simulink model "FuelPrimary_harness"  (Simulink 7.7)
settings: Solver=FixedStepDiscrete  SolverMode=SingleTasking  StartTime=0.0  StopTime=100  FixedStep=srate  RelTol=1e-3
InitFcn:
  | if signalbuilder('FuelPrimary_harness/Signal_Builder','activegroup') == 10
  |   CD_FUEL_PRIMARY_FUNCTION.DataType = 'uint8';
  |   CD_FUEL_PRIMARY_FUNCTION.Value = 255;
  | 
  | else
  |   CD_FUEL_PRIMARY_FUNCTION.DataType = 'uint8';
  |   CD_FUEL_PRIMARY_FUNCTION.Value = 0;
  | end
  | 
  | if signalbuilder('FuelPrimary_harness/Signal_Builder','activegroup') == 7
  |   CD_FUEL_PRIMARY_ON_SECONDARY_FAILURE.DataType = 'uint8';
  |   CD_FUEL_PRIMARY_ON_SECONDARY_FAILURE.Value = 0;
  | else
  |   CD_FUEL_PRIMARY_ON_SECONDARY_FAILURE.DataType = 'uint8';
  |   CD_FUEL_PRIMARY_ON_SECONDARY_FAILURE.Value = 255;
  | end
  | 
  | if signalbuilder('FuelPrimary_harness/Signal_Builder','activegroup') == 11
  |   CD_FUEL_PRIMARY_FEEDBACK_FUNCTION.DataType = 'uint8';
  |   CD_FUEL_PRIMARY_FEEDBACK_FUNCTION.Value = 255;
  | elseif signalbuilder('FuelPrimary_harness/Signal_Builder','activegroup') == 10
  |   CD_FUEL_PRIMARY_FEEDBACK_FUNCTION.DataType = 'uint8';
  |   CD_FUEL_PRIMARY_FEEDBACK_FUNCTION.Value = 255;
  | else
  |   CD_FUEL_PRIMARY_FEEDBACK_FUNCTION.DataType = 'uint8';
  |   CD_FUEL_PRIMARY_FEEDBACK_FUNCTION.Value = 0;
  | end
  | 
  | if signalbuilder('FuelPrimary_harness/Signal_Builder','activegroup') == 12
  |   CD_NO_FUEL_WITH_LOW_EOP_FUNCTION.DataType = 'uint8';
  |   CD_NO_FUEL_WITH_LOW_EOP_FUNCTION.Value = 0;
  | elseif signalbuilder('FuelPrimary_harness/Signal_Builder','activegroup') == 13
  |   CD_NO_FUEL_WITH_LOW_EOP_FUNCTION.DataType = 'uint8';
  |   CD_NO_FUEL_WITH_LOW_EOP_FUNCTION.Value = 0;
  | else
  | CD_NO_FUEL_WITH_LOW_EOP_FUNCTION.DataType = 'uint8';
  |   CD_NO_FUEL_WITH_LOW_EOP_FUNCTION.Value = 255;
  | end
  | 
  | 
  | 
  | if signalbuilder('FuelPrimary_harness/Signal_Builder','activegroup') == 13
  |   CD_EOP_FUNCTION.DataType = 'uint8';
  |   CD_EOP_FUNCTION.Value = 1;
  | else
  |   CD_EOP_FUNCTION.DataType = 'uint8';
  |   CD_EOP_FUNCTION.Value = 0;
  | end
undefined symbols (not defined in the file): ACTIVE, ENGINE_CRANKING, ENGINE_NOT_RUNNING, FAILURE, INACTIVE, MXGTW_FUEL_PULL_TIME, NON_FUNCTIONAL, NORMAL, OORL, sigbuilder_block, UNLIMITED
libraries: simulink x2, MX_Library x1
CloseFcn:
  | rtwprivate ssgencode ModelCloseRequest sle_main_controller
settings Model: Creator=smindema  LastModifiedBy=aliebel  RecordCoverage=on  CovPath=Fuel_Primary_Relay/RelaySolenoid  CovMetricSettings=dcmt  CovHTMLOptions=-aTS=1 -bRG=1 -bTC=1 -hTR=0 -nFC=0 -scm=1 -bcm=1 -xEv=0  CovForceBlockReductionOff=off  covSaveCumulativeToWorkspaceVar=off  CovModelRefEnable=off
settings MATStruct: SampleTime=0.01  Offset=0  Priority=[1.0]
settings DataIOCC: LimitDataPoints=off  SaveOutput=off  SaveTime=off
settings OptimizationCC: BlockReduction=off  InlineParams=on  ExpressionFolding=off  StateBitsets=on  DataBitsets=on  UseTempVars=on  InitFltsAndDblsToZero=on  NoFixptDivByZeroProtection=on  EfficientFloat2IntCast=on  OptimizeModelRefInitCode=on
settings DebuggingCC: SaveWithParameterizedLinksMsg=none  MultiTaskDSMMsg=warning  MultiTaskCondExecSysMsg=none  IntegerOverflowMsg=none  ModelReferenceCSMismatchMessage=warning
settings HardwareCC: ProdBitPerInt=16  ProdBitPerPointer=16  ProdIntDivRoundTo=Floor  ProdEndianess=BigEndian  ProdWordSize=16  ProdHWDeviceType=Motorola HC12
settings ModelReferenceCC: ModelReferenceNumInstancesAllowed=Single
settings RTWCC: SystemTargetFile=ert.tlc  GenCodeOnly=on  TemplateMakefile=ert_default_tmf  Description=Real-Time Workshop Embedded Coder (no auto configuration)  GenerateReport=on  RetainRTWFile=on  ProcessScript=ert_make_rtw_hook  IncludeHyperlinkInReport=on  LaunchReport=on  IncludeERTFirstTime=on
settings RTWCC: CustomHeaderCode=|
  | #include "cpp_req_defines.h"
  | #include "hw_fin.h"
  | #include "cdata.h"
settings CodeAppCC: IgnoreCustomStorageClasses=off  DefineNamingRule=UpperCase
settings ERTTargetCC: TargetFcnLib=ansi_tfl_tmw.mat  FunctionExecutionProfile=off  MultiwordLength=2048  GenerateSampleERTMain=on  IncludeMdlTerminateFcn=off  SupportAbsoluteTime=off  SupportNonFinite=off  SupportComplex=off  PurelyIntegerCode=on  ERTCustomFileTemplate=gen_rtw_req_defines_h.tlc  GlobalDataDefinition=InSeparateSourceFile  GlobalDataReference=InSeparateHeaderFile  ConvertIfToSwitch=off

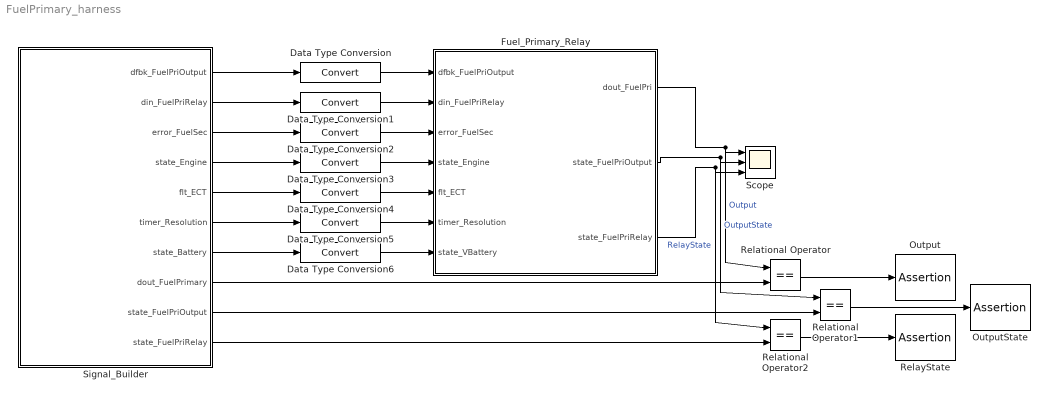
== system FuelPrimary_harness ==
  Data Type Conversion{,1..6} (7 alike) : DataTypeConversion
  Fuel_Primary_Relay : Subsystem  TreatAsAtomicUnit=on
      settings: RTWSystemCode=Function  RTWFcnNameOpts=Use subsystem name
  Output : Assertion  Enabled=off
  OutputState : Assertion  Enabled=off
  Relational Operator : RelationalOperator  Operator===  OutDataTypeStr=boolean
  Relational Operator1 : RelationalOperator  Operator===  OutDataTypeStr=boolean
  Relational Operator2 : RelationalOperator  Operator===  OutDataTypeStr=boolean
  RelayState : Assertion  Enabled=off
  Scope : Scope  NumInputPorts=3
      settings: YMin=0~0~0  YMax=2~10~10  MaxDataPoints=50000
  Signal_Builder : Subsystem  Tag=STV Subsys  LoadFcn=sigbuilder_block('load');  StartFcn=sigbuilder_block('start');  StopFcn=sigbuilder_block('stop');  ClipboardFcn=sigbuilder_block('clipboard');  mask(Sigbuilder block){}
      mask help: Sigbuilder GUI
      mask init:
      | if ~strcmp(get_param(bdroot(gcbh),'SimulationStatus'),'stopped') tuvar = sigbuilder_block('maskInit'); end
      settings: CopyFcn=sigbuilder_block('copy');  DeleteFcn=sigbuilder_block('delete');  ModelCloseFcn=sigbuilder_block('modelClose');  PreSaveFcn=sigbuilder_block('preSave');  NameChangeFcn=sigbuilder_block('namechange');  OpenFcn=sigbuilder_block('open',[55.5 123.75 1080 620.25 ]);  CloseFcn=sigbuilder_block('close');
      mask Display: plot(0,0,100,100,[10,10,40,40,10],[80,20,20,80,80],[40,10],[50,50], [40,27,10],[65,72,56],[40,25,25,10],[28,28,43,43]);
  wires:
  Fuel_Primary_Relay/1(dout_FuelPri) -> Scope/1, Relational Operator/1  "Output"
  Fuel_Primary_Relay/2(state_FuelPriOutput) -> Scope/2, Relational Operator1/1  "OutputState"
  Fuel_Primary_Relay/3(state_FuelPriRelay) -> Scope/3, Relational Operator2/1  "RelayState"
  Relational Operator/1 -> Output/1
  Relational Operator1/1 -> OutputState/1
  Relational Operator2/1 -> RelayState/1
  Signal_Builder/8(dout_FuelPrimary) -> Relational Operator/2
  Signal_Builder/9(state_FuelPriOutput) -> Relational Operator1/2
  Signal_Builder/10(state_FuelPriRelay) -> Relational Operator2/2
  Data Type Conversion/1 -> Fuel_Primary_Relay/1(dfbk_FuelPriOutput)
  Data Type Conversion1/1 -> Fuel_Primary_Relay/2(din_FuelPriRelay)
  Data Type Conversion2/1 -> Fuel_Primary_Relay/3(error_FuelSec)
  Data Type Conversion3/1 -> Fuel_Primary_Relay/4(state_Engine)
  Data Type Conversion4/1 -> Fuel_Primary_Relay/5(flt_ECT)
  Data Type Conversion5/1 -> Fuel_Primary_Relay/6(timer_Resolution)
  Data Type Conversion6/1 -> Fuel_Primary_Relay/7(state_VBattery)
  Signal_Builder/1(dfbk_FuelPriOutput) -> Data Type Conversion/1
  Signal_Builder/2(din_FuelPriRelay) -> Data Type Conversion1/1
  Signal_Builder/3(error_FuelSec) -> Data Type Conversion2/1
  Signal_Builder/4(state_Engine) -> Data Type Conversion3/1
  Signal_Builder/5(flt_ECT) -> Data Type Conversion4/1
  Signal_Builder/6(timer_Resolution) -> Data Type Conversion5/1
  Signal_Builder/7(state_Battery) -> Data Type Conversion6/1

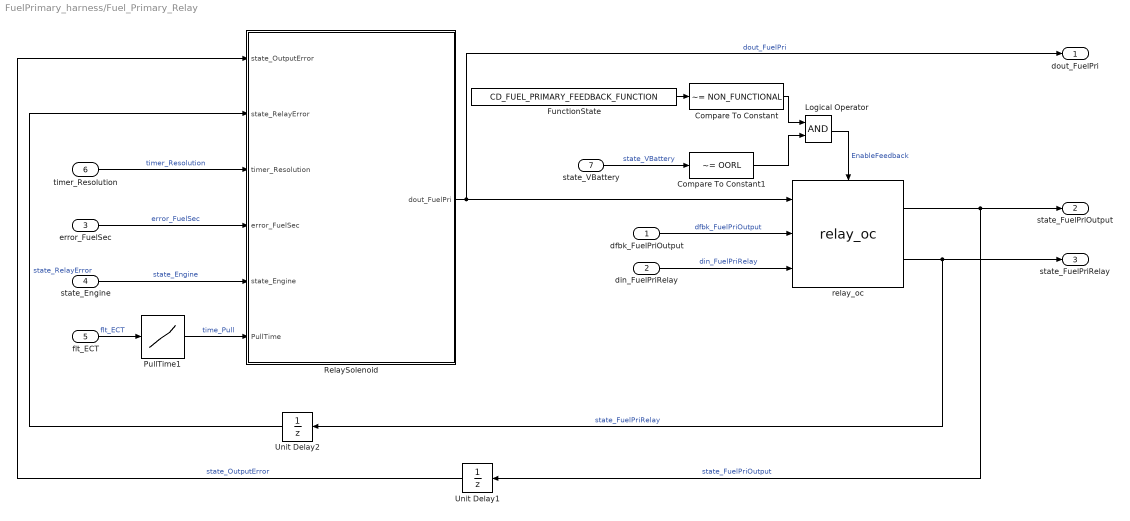
== system FuelPrimary_harness/Fuel_Primary_Relay ==
  dfbk_FuelPriOutput : Inport  OutDataTypeStr=boolean
  din_FuelPriRelay : Inport  Port=2  OutDataTypeStr=boolean
  error_FuelSec : Inport  Port=3  OutDataTypeStr=uint8
  state_Engine : Inport  Port=4
  flt_ECT : Inport  Port=5  OutDataTypeStr=uint16
  timer_Resolution : Inport  Port=6  OutDataTypeStr=uint8
  state_VBattery : Inport  Port=7
  Compare To Constant : simulink/Logic and Bit Operations/Compare To Constant  SystemSampleTime=-1  relop=~=  const=NON_FUNCTIONAL  LogicOutDataTypeMode=boolean  ZeroCross=off
  Compare To Constant1 : simulink/Logic and Bit Operations/Compare To Constant  SystemSampleTime=-1  relop=~=  const=OORL  LogicOutDataTypeMode=boolean  ZeroCross=off
  FunctionState : Constant  Value=CD_FUEL_PRIMARY_FEEDBACK_FUNCTION  OutDataTypeStr=uint8
  Logical Operator : Logic  AllPortsSameDT=off  OutDataTypeStr=boolean
  PullTime1 : Lookup  InputValues=0:8:336  Table=MXGTW_FUEL_PULL_TIME  LookUpMeth=Use Input Nearest  OutDataTypeStr=uint16  RndMeth=Nearest
      settings: AttributesFormatString=input = %<InputValues>\noutput = %<OutputValues>\nlookup = %<LookUpMeth>\nrounding = %<RndMeth>
  RelaySolenoid : Stateflow chart  TreatAsAtomicUnit=on
  Unit Delay1 : UnitDelay  SampleTime=-1
      settings: AttributesFormatString=<initial=%<X0>>\n<tsample=%<SampleTime>>
  Unit Delay2 : UnitDelay  SampleTime=-1
      settings: AttributesFormatString=<initial=%<X0>>\n<tsample=%<SampleTime>>
  relay_oc : MX_Library/relay_oc  SystemSampleTime=-1  ERROR_ON_DB_CNT=CD_FUEL_PRIMARY_DEBOUNCE_ERROR_ON  ERROR_OFF_DB_CNT=CD_FUEL_PRIMARY_DEBOUNCE_ERROR_OFF  NORMAL_DB_CNT=CD_FUEL_PRIMARY_DEBOUNCE_NORMAL
  dout_FuelPri : Outport  OutDataTypeStr=boolean
  state_FuelPriOutput : Outport  Port=2  OutDataTypeStr=uint8
  state_FuelPriRelay : Outport  Port=3  OutDataTypeStr=uint8
  wires:
  timer_Resolution/1 -> RelaySolenoid/3(timer_Resolution)  "timer_Resolution"
  flt_ECT/1 -> PullTime1/1  "flt_ECT"
  state_Engine/1 -> RelaySolenoid/5(state_Engine)  "state_Engine"
  Logical Operator/1 -> relay_oc/Enable  "EnableFeedback"
  Compare To Constant1/1 -> Logical Operator/2
  Compare To Constant/1 -> Logical Operator/1
  state_VBattery/1 -> Compare To Constant1/1  "state_VBattery"
  FunctionState/1 -> Compare To Constant/1
  relay_oc/1 -> Unit Delay1/1, state_FuelPriOutput/1  "state_FuelPriOutput"
  Unit Delay2/1 -> RelaySolenoid/2(state_RelayError)  "state_RelayError"
  Unit Delay1/1 -> RelaySolenoid/1(state_OutputError)  "state_OutputError"
  relay_oc/2 -> Unit Delay2/1, state_FuelPriRelay/1  "state_FuelPriRelay"
  din_FuelPriRelay/1 -> relay_oc/3  "din_FuelPriRelay"
  dfbk_FuelPriOutput/1 -> relay_oc/2  "dfbk_FuelPriOutput"
  RelaySolenoid/1(dout_FuelPri) -> dout_FuelPri/1, relay_oc/1  "dout_FuelPri"
  error_FuelSec/1 -> RelaySolenoid/4(error_FuelSec)  "error_FuelSec"
  PullTime1/1 -> RelaySolenoid/6(PullTime)  "time_Pull"

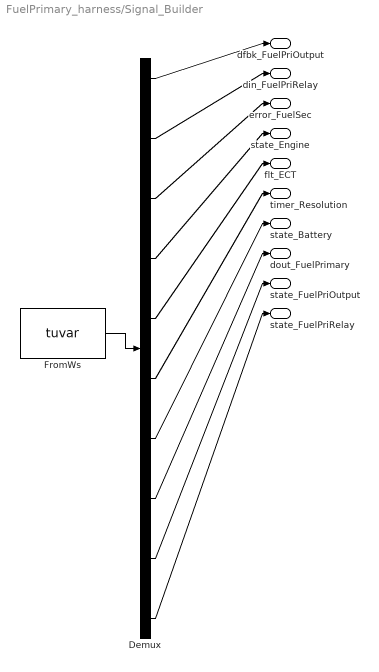
== system FuelPrimary_harness/Signal_Builder ==
  Demux : Demux  Tag=STV Demux  Outputs=10
  FromWs : FromWorkspace  Tag=STV FromWs  VariableName=tuvar  SampleTime=0  SigBuilderData=DataTag0  VnvData=DataTag1
      SigBuilderData=|
      | common.afterFinalStr = 'Extrapolate'
      | common.sampleTime = 0
      | dataSet(1).timeRange = [0 100]
      | dataSet(1).name = 'Normal'
      | dataSet(2).timeRange = [0 100]
      | dataSet(2).name = 'Relay OC'
      | dataSet(3).timeRange = [0 100]
      | dataSet(3).name = 'Output Cont Error'
      | dataSet(4).timeRange = [0 100]
      | dataSet(4).name = 'Relay Error On'
      | dataSet(5).timeRange = [0 100]
      | dataSet(5).name = 'Relay Error Off'
      | dataSet(6).timeRange = [0 100]
      | dataSet(6).name = 'Battery'
      | dataSet(7).timeRange = [0 100]
      | dataSet(7).name = 'SecondaryFuel'
      | dataSet(8).timeRange = [0 100]
      | dataSet(8).name = 'Error ON'
      | dataSet(9).timeRange = [0 100]
      | dataSet(9).name = 'Error OFF'
      | dataSet(10).timeRange = [0 100]
      | dataSet(10).name = 'NONFUNC'
      | dataSet(11).timeRange = [0 100]
      | dataSet(11).name = 'NO FDBK'
      | dataSet(12).timeRange = [0 100]
      | dataSet(12).name = 'Output Error On'
      | dataSet(13).timeRange = [0 100]
      | dataSet(13).name = 'Output Error Off'
      | sbobj.Groups(1).Name = 'Normal'
      | sbobj.Groups(1).Signals(1).Name = 'dfbk_FuelPriOutput'
      | sbobj.Groups(1).Signals(1).XData = [0 20 20 22.2 22.2 60 60 61.4 61.4 100]
      | sbobj.Groups(1).Signals(1).YData = [0 0 1 1 0 0 1 1 0 0]
      | sbobj.Groups(1).Signals(2).Name = 'din_FuelPriRelay'
      | sbobj.Groups(1).Signals(2).XData = [0 20 20 22.2 22.2 60 60 61.4 61.4 100]
      | sbobj.Groups(1).Signals(2).YData = [0 0 1 1 0 0 1 1 0 0]
      | sbobj.Groups(1).Signals(3).Name = 'error_FuelSec'
      | sbobj.Groups(1).Signals(3).XData = [0 100]
      | sbobj.Groups(1).Signals(3).YData = [8 8]
      | sbobj.Groups(1).Signals(4).Name = 'state_Engine'
      | sbobj.Groups(1).Signals(4).XData = [0 20 20 30 30 50 50 60 60 61.2 61.2 62.6 62.6 64.2 64.2 100]
      | sbobj.Groups(1).Signals(4).YData = [1 1 2 2 3 3 1 1 2 2 1 1 2 2 1 1]
      | sbobj.Groups(1).Signals(5).Name = 'flt_ECT'
      | sbobj.Groups(1).Signals(5).XData = [0 49.9 49.9 100]
      | sbobj.Groups(1).Signals(5).YData = [0 0 200 200]
      | sbobj.Groups(1).Signals(6).Name = 'timer_Resolution'
      | sbobj.Groups(1).Signals(6).XData = [0 61.5 61.5 64.8 64.8 100]
      | sbobj.Groups(1).Signals(6).YData = [0 0 1 1 0 0]
      | sbobj.Groups(1).Signals(7).Name = 'state_Battery'
      | sbobj.Groups(1).Signals(7).XData = [0 100]
      | sbobj.Groups(1).Signals(7).YData = [8 8]
      | sbobj.Groups(1).Signals(8).Name = 'dout_FuelPrimary'
      | sbobj.Groups(1).Signals(8).XData = [0 20 20 22.11 22.11 60 60 61.2 61.2 100]
      | sbobj.Groups(1).Signals(8).YData = [0 0 1 1 0 0 1 1 0 0]
      | sbobj.Groups(1).Signals(9).Name = 'state_FuelPriOutput'
      | sbobj.Groups(1).Signals(9).XData = [0 100]
      | sbobj.Groups(1).Signals(9).YData = [8 8]
      | sbobj.Groups(1).Signals(10).Name = 'state_FuelPriRelay'
      | sbobj.Groups(1).Signals(10).XData = [0 100]
      | sbobj.Groups(1).Signals(10).YData = [8 8]
      | sbobj.Groups(2).Name = 'Relay OC'
      | sbobj.Groups(2).Signals(1).Name = 'dfbk_FuelPriOutput'
      | sbobj.Groups(2).Signals(1).XData = [0 10 10 30 30 100]
      | sbobj.Groups(2).Signals(1).YData = [0 0 1 1 0 0]
      | sbobj.Groups(2).Signals(2).Name = 'din_FuelPriRelay'
      | sbobj.Groups(2).Signals(2).XData = [0 100]
      | sbobj.Groups(2).Signals(2).YData = [0 0]
      | sbobj.Groups(2).Signals(3).Name = 'error_FuelSec'
      | sbobj.Groups(2).Signals(3).XData = [0 100]
      | sbobj.Groups(2).Signals(3).YData = [8 8]
      | sbobj.Groups(2).Signals(4).Name = 'state_Engine'
      | sbobj.Groups(2).Signals(4).XData = [0 20 20 30 30 50 50 69.9 100]
      | sbobj.Groups(2).Signals(4).YData = [1 1 2 2 3 3 1 1 1]
      | sbobj.Groups(2).Signals(5).Name = 'flt_ECT'
      | sbobj.Groups(2).Signals(5).XData = [0 100]
      | sbobj.Groups(2).Signals(5).YData = [150 150]
      | sbobj.Groups(2).Signals(6).Name = 'timer_Resolution'
      | sbobj.Groups(2).Signals(6).XData = [0 100]
      | sbobj.Groups(2).Signals(6).YData = [0 0]
      | sbobj.Groups(2).Signals(7).Name = 'state_Battery'
      | sbobj.Groups(2).Signals(7).XData = [0 100]
      | sbobj.Groups(2).Signals(7).YData = [8 8]
      | sbobj.Groups(2).Signals(8).Name = 'dout_FuelPrimary'
      | sbobj.Groups(2).Signals(8).XData = [0 100]
      | sbobj.Groups(2).Signals(8).YData = [0 0]
      | sbobj.Groups(2).Signals(9).Name = 'state_FuelPriOutput'
      | sbobj.Groups(2).Signals(9).XData = [0 10.05 10.05 100]
      | sbobj.Groups(2).Signals(9).YData = [8 8 7 7]
      | sbobj.Groups(2).Signals(10).Name = 'state_FuelPriRelay'
      | sbobj.Groups(2).Signals(10).XData = [0 10.05 100]
      | sbobj.Groups(2).Signals(10).YData = [8 8 8]
      | sbobj.Groups(3).Name = 'Output Cont Error'
      | sbobj.Groups(3).Signals(1).Name = 'dfbk_FuelPriOutput'
      | sbobj.Groups(3).Signals(1).XData = [0 100]
      | sbobj.Groups(3).Signals(1).YData = [0 0]
      | sbobj.Groups(3).Signals(2).Name = 'din_FuelPriRelay'
      | sbobj.Groups(3).Signals(2).XData = [0 20 20 21.61 21.61 60 60 61.61 61.61 100]
      | sbobj.Groups(3).Signals(2).YData = [0 0 1 1 0 0 1 1 0 0]
      | sbobj.Groups(3).Signals(3).Name = 'error_FuelSec'
      | sbobj.Groups(3).Signals(3).XData = [0 100]
      | sbobj.Groups(3).Signals(3).YData = [8 8]
      | sbobj.Groups(3).Signals(4).Name = 'state_Engine'
      | sbobj.Groups(3).Signals(4).XData = [0 20 20 30 30 50 50 60 60 70.1 70.1 80.1 100]
      | sbobj.Groups(3).Signals(4).YData = [1 1 2 2 3 3 1 1 2 2 1 1 1]
      | sbobj.Groups(3).Signals(5).Name = 'flt_ECT'
      | sbobj.Groups(3).Signals(5).XData = [0 100]
      | sbobj.Groups(3).Signals(5).YData = [130 130]
      | sbobj.Groups(3).Signals(6).Name = 'timer_Resolution'
      | sbobj.Groups(3).Signals(6).XData = [0 100]
      | sbobj.Groups(3).Signals(6).YData = [0 0]
      | sbobj.Groups(3).Signals(7).Name = 'state_Battery'
      | sbobj.Groups(3).Signals(7).XData = [0 100]
      | sbobj.Groups(3).Signals(7).YData = [8 8]
      | sbobj.Groups(3).Signals(8).Name = 'dout_FuelPrimary'
      | sbobj.Groups(3).Signals(8).XData = [0 20 20 21.61 21.61 60 60 61.61 61.61 100]
      | sbobj.Groups(3).Signals(8).YData = [0 0 1 1 0 0 1 1 0 0]
      | sbobj.Groups(3).Signals(9).Name = 'state_FuelPriOutput'
      | sbobj.Groups(3).Signals(9).XData = [0 20.05 20.05 100]
      | sbobj.Groups(3).Signals(9).YData = [8 8 28 28]
      | sbobj.Groups(3).Signals(10).Name = 'state_FuelPriRelay'
      | sbobj.Groups(3).Signals(10).XData = [0 100]
      | sbobj.Groups(3).Signals(10).YData = [8 8]
      | sbobj.Groups(4).Name = 'Relay Error On'
      | sbobj.Groups(4).Signals(1).Name = 'dfbk_FuelPriOutput'
      | sbobj.Groups(4).Signals(1).XData = [0 100]
      | sbobj.Groups(4).Signals(1).YData = [0 0]
      | sbobj.Groups(4).Signals(2).Name = 'din_FuelPriRelay'
      | sbobj.Groups(4).Signals(2).XData = [0 10 10 30 30 100]
      | sbobj.Groups(4).Signals(2).YData = [0 0 1 1 0 0]
      | sbobj.Groups(4).Signals(3).Name = 'error_FuelSec'
      | sbobj.Groups(4).Signals(3).XData = [0 100]
      | sbobj.Groups(4).Signals(3).YData = [8 8]
      | sbobj.Groups(4).Signals(4).Name = 'state_Engine'
      | sbobj.Groups(4).Signals(4).XData = [0 20 20 30 30 50 50 69.9 100]
      | sbobj.Groups(4).Signals(4).YData = [1 1 2 2 3 3 1 1 1]
      | sbobj.Groups(4).Signals(5).Name = 'flt_ECT'
      | sbobj.Groups(4).Signals(5).XData = [0 100]
      | sbobj.Groups(4).Signals(5).YData = [0 0]
      | sbobj.Groups(4).Signals(6).Name = 'timer_Resolution'
      | sbobj.Groups(4).Signals(6).XData = [0 100]
      | sbobj.Groups(4).Signals(6).YData = [0 0]
      | sbobj.Groups(4).Signals(7).Name = 'state_Battery'
      | sbobj.Groups(4).Signals(7).XData = [0 100]
      | sbobj.Groups(4).Signals(7).YData = [8 8]
      | sbobj.Groups(4).Signals(8).Name = 'dout_FuelPrimary'
      | sbobj.Groups(4).Signals(8).XData = [0 100]
      | sbobj.Groups(4).Signals(8).YData = [0 0]
      | sbobj.Groups(4).Signals(9).Name = 'state_FuelPriOutput'
      | sbobj.Groups(4).Signals(9).XData = [0 100]
      | sbobj.Groups(4).Signals(9).YData = [8 8]
      | sbobj.Groups(4).Signals(10).Name = 'state_FuelPriRelay'
      | sbobj.Groups(4).Signals(10).XData = [0 10.51 10.51 100]
      | sbobj.Groups(4).Signals(10).YData = [8 8 2 2]
      | sbobj.Groups(5).Name = 'Relay Error Off'
      | sbobj.Groups(5).Signals(1).Name = 'dfbk_FuelPriOutput'
      | sbobj.Groups(5).Signals(1).XData = [0 20 20 30.5 30.5 100]
      | sbobj.Groups(5).Signals(1).YData = [0 0 1 1 0 0]
      | sbobj.Groups(5).Signals(2).Name = 'din_FuelPriRelay'
      | sbobj.Groups(5).Signals(2).XData = [0 100]
      | sbobj.Groups(5).Signals(2).YData = [0 0]
      | sbobj.Groups(5).Signals(3).Name = 'error_FuelSec'
      | sbobj.Groups(5).Signals(3).XData = [0 100]
      | sbobj.Groups(5).Signals(3).YData = [8 8]
      | sbobj.Groups(5).Signals(4).Name = 'state_Engine'
      | sbobj.Groups(5).Signals(4).XData = [0 20 20 30 30 50 50 69.9 100]
      | sbobj.Groups(5).Signals(4).YData = [1 1 2 2 3 3 1 1 1]
      | sbobj.Groups(5).Signals(5).Name = 'flt_ECT'
      | sbobj.Groups(5).Signals(5).XData = [0 100]
      | sbobj.Groups(5).Signals(5).YData = [340 340]
      | sbobj.Groups(5).Signals(6).Name = 'timer_Resolution'
      | sbobj.Groups(5).Signals(6).XData = [0 100]
      | sbobj.Groups(5).Signals(6).YData = [0 0]
      | sbobj.Groups(5).Signals(7).Name = 'state_Battery'
      | sbobj.Groups(5).Signals(7).XData = [0 100]
      | sbobj.Groups(5).Signals(7).YData = [8 8]
      | sbobj.Groups(5).Signals(8).Name = 'dout_FuelPrimary'
      | sbobj.Groups(5).Signals(8).XData = [0 20 20 20.06 20.06 100]
      | sbobj.Groups(5).Signals(8).YData = [0 0 1 1 0 0]
      | sbobj.Groups(5).Signals(9).Name = 'state_FuelPriOutput'
      | sbobj.Groups(5).Signals(9).XData = [0 100]
      | sbobj.Groups(5).Signals(9).YData = [8 8]
      | sbobj.Groups(5).Signals(10).Name = 'state_FuelPriRelay'
      | sbobj.Groups(5).Signals(10).XData = [0 20.05 20.05 100]
      | sbobj.Groups(5).Signals(10).YData = [8 8 3 3]
      | sbobj.Groups(6).Name = 'Battery'
      | sbobj.Groups(6).Signals(1).Name = 'dfbk_FuelPriOutput'
      | sbobj.Groups(6).Signals(1).XData = [0 20 20 21 21 100]
      | sbobj.Groups(6).Signals(1).YData = [0 0 1 1 0 0]
      | sbobj.Groups(6).Signals(2).Name = 'din_FuelPriRelay'
      | sbobj.Groups(6).Signals(2).XData = [0 20 20 21 21 100]
      | sbobj.Groups(6).Signals(2).YData = [0 0 1 1 0 0]
      | sbobj.Groups(6).Signals(3).Name = 'error_FuelSec'
      | sbobj.Groups(6).Signals(3).XData = [0 100]
      | sbobj.Groups(6).Signals(3).YData = [8 8]
      | sbobj.Groups(6).Signals(4).Name = 'state_Engine'
      | sbobj.Groups(6).Signals(4).XData = [0 20 20 30 30 50 50 69.9 100]
      | sbobj.Groups(6).Signals(4).YData = [1 1 2 2 3 3 1 1 1]
      | sbobj.Groups(6).Signals(5).Name = 'flt_ECT'
      | sbobj.Groups(6).Signals(5).XData = [0 100]
      | sbobj.Groups(6).Signals(5).YData = [340 340]
      | sbobj.Groups(6).Signals(6).Name = 'timer_Resolution'
      | sbobj.Groups(6).Signals(6).XData = [0 100]
      | sbobj.Groups(6).Signals(6).YData = [0 0]
      | sbobj.Groups(6).Signals(7).Name = 'state_Battery'
      | sbobj.Groups(6).Signals(7).XData = [0 100]
      | sbobj.Groups(6).Signals(7).YData = [22 22]
      | sbobj.Groups(6).Signals(8).Name = 'dout_FuelPrimary'
      | sbobj.Groups(6).Signals(8).XData = [0 20 20 20.91 20.91 100]
      | sbobj.Groups(6).Signals(8).YData = [0 0 1 1 0 0]
      | sbobj.Groups(6).Signals(9).Name = 'state_FuelPriOutput'
      | sbobj.Groups(6).Signals(9).XData = [0 100]
      | sbobj.Groups(6).Signals(9).YData = [8 8]
      | sbobj.Groups(6).Signals(10).Name = 'state_FuelPriRelay'
      | sbobj.Groups(6).Signals(10).XData = [0 100]
      | sbobj.Groups(6).Signals(10).YData = [8 8]
      | sbobj.Groups(7).Name = 'SecondaryFuel'
      | sbobj.Groups(7).Signals(1).Name = 'dfbk_FuelPriOutput'
      | sbobj.Groups(7).Signals(1).XData = [0 20 20 50 50 100]
      | sbobj.Groups(7).Signals(1).YData = [0 0 1 1 0 0]
      | sbobj.Groups(7).Signals(2).Name = 'din_FuelPriRelay'
      | sbobj.Groups(7).Signals(2).XData = [0 20 20 50 50 100]
      | sbobj.Groups(7).Signals(2).YData = [0 0 1 1 0 0]
      | sbobj.Groups(7).Signals(3).Name = 'error_FuelSec'
      | sbobj.Groups(7).Signals(3).XData = [0 100]
      | sbobj.Groups(7).Signals(3).YData = [22 22]
      | sbobj.Groups(7).Signals(4).Name = 'state_Engine'
      | sbobj.Groups(7).Signals(4).XData = [0 20 20 30 30 50 50 69.9 100]
      | sbobj.Groups(7).Signals(4).YData = [1 1 2 2 3 3 1 1 1]
      | sbobj.Groups(7).Signals(5).Name = 'flt_ECT'
      | sbobj.Groups(7).Signals(5).XData = [0 100]
      | sbobj.Groups(7).Signals(5).YData = [0 0]
      | sbobj.Groups(7).Signals(6).Name = 'timer_Resolution'
      | sbobj.Groups(7).Signals(6).XData = [0 100]
      | sbobj.Groups(7).Signals(6).YData = [0 0]
      | sbobj.Groups(7).Signals(7).Name = 'state_Battery'
      | sbobj.Groups(7).Signals(7).XData = [0 100]
      | sbobj.Groups(7).Signals(7).YData = [8 8]
      | sbobj.Groups(7).Signals(8).Name = 'dout_FuelPrimary'
      | sbobj.Groups(7).Signals(8).XData = [0 20 20 50 50 100]
      | sbobj.Groups(7).Signals(8).YData = [0 0 1 1 0 0]
      | sbobj.Groups(7).Signals(9).Name = 'state_FuelPriOutput'
      | sbobj.Groups(7).Signals(9).XData = [0 100]
      | sbobj.Groups(7).Signals(9).YData = [8 8]
      | sbobj.Groups(7).Signals(10).Name = 'state_FuelPriRelay'
      | sbobj.Groups(7).Signals(10).XData = [0 100]
      | sbobj.Groups(7).Signals(10).YData = [8 8]
      | sbobj.Groups(8).Name = 'Error ON'
      | sbobj.Groups(8).Signals(1).Name = 'dfbk_FuelPriOutput'
      | sbobj.Groups(8).Signals(1).XData = [0 10 10 30 30 100]
      | sbobj.Groups(8).Signals(1).YData = [0 0 1 1 0 0]
      | sbobj.Groups(8).Signals(2).Name = 'din_FuelPriRelay'
      | sbobj.Groups(8).Signals(2).XData = [0 10 10 30 30 100]
      | sbobj.Groups(8).Signals(2).YData = [0 0 1 1 0 0]
      | sbobj.Groups(8).Signals(3).Name = 'error_FuelSec'
      | sbobj.Groups(8).Signals(3).XData = [0 100]
      | sbobj.Groups(8).Signals(3).YData = [8 8]
      | sbobj.Groups(8).Signals(4).Name = 'state_Engine'
      | sbobj.Groups(8).Signals(4).XData = [0 20 20 30 30 50 50 69.9 100]
      | sbobj.Groups(8).Signals(4).YData = [1 1 2 2 3 3 1 1 1]
      | sbobj.Groups(8).Signals(5).Name = 'flt_ECT'
      | sbobj.Groups(8).Signals(5).XData = [0 100]
      | sbobj.Groups(8).Signals(5).YData = [150 150]
      | sbobj.Groups(8).Signals(6).Name = 'timer_Resolution'
      | sbobj.Groups(8).Signals(6).XData = [0 100]
      | sbobj.Groups(8).Signals(6).YData = [0 0]
      | sbobj.Groups(8).Signals(7).Name = 'state_Battery'
      | sbobj.Groups(8).Signals(7).XData = [0 100]
      | sbobj.Groups(8).Signals(7).YData = [8 8]
      | sbobj.Groups(8).Signals(8).Name = 'dout_FuelPrimary'
      | sbobj.Groups(8).Signals(8).XData = [0 100]
      | sbobj.Groups(8).Signals(8).YData = [0 0]
      | sbobj.Groups(8).Signals(9).Name = 'state_FuelPriOutput'
      | sbobj.Groups(8).Signals(9).XData = [0 10.51 10.51 100]
      | sbobj.Groups(8).Signals(9).YData = [8 8 2 2]
      | sbobj.Groups(8).Signals(10).Name = 'state_FuelPriRelay'
      | sbobj.Groups(8).Signals(10).XData = [0 15.1 100]
      | sbobj.Groups(8).Signals(10).YData = [8 8 8]
      | sbobj.Groups(9).Name = 'Error OFF'
      | sbobj.Groups(9).Signals(1).Name = 'dfbk_FuelPriOutput'
      | sbobj.Groups(9).Signals(1).XData = [0 10 30 100]
      | sbobj.Groups(9).Signals(1).YData = [0 0 0 0]
      | sbobj.Groups(9).Signals(2).Name = 'din_FuelPriRelay'
      | sbobj.Groups(9).Signals(2).XData = [0 10 30 100]
      | sbobj.Groups(9).Signals(2).YData = [0 0 0 0]
      | sbobj.Groups(9).Signals(3).Name = 'error_FuelSec'
      | sbobj.Groups(9).Signals(3).XData = [0 100]
      | sbobj.Groups(9).Signals(3).YData = [8 8]
      | sbobj.Groups(9).Signals(4).Name = 'state_Engine'
      | sbobj.Groups(9).Signals(4).XData = [0 20 20 30 30 50 50 69.9 100]
      | sbobj.Groups(9).Signals(4).YData = [1 1 2 2 3 3 1 1 1]
      | sbobj.Groups(9).Signals(5).Name = 'flt_ECT'
      | sbobj.Groups(9).Signals(5).XData = [0 100]
      | sbobj.Groups(9).Signals(5).YData = [150 150]
      | sbobj.Groups(9).Signals(6).Name = 'timer_Resolution'
      | sbobj.Groups(9).Signals(6).XData = [0 100]
      | sbobj.Groups(9).Signals(6).YData = [0 0]
      | sbobj.Groups(9).Signals(7).Name = 'state_Battery'
      | sbobj.Groups(9).Signals(7).XData = [0 100]
      | sbobj.Groups(9).Signals(7).YData = [8 8]
      | sbobj.Groups(9).Signals(8).Name = 'dout_FuelPrimary'
      | sbobj.Groups(9).Signals(8).XData = [0 20 20 20.06 20.06 100]
      | sbobj.Groups(9).Signals(8).YData = [0 0 1 1 0 0]
      | sbobj.Groups(9).Signals(9).Name = 'state_FuelPriOutput'
      | sbobj.Groups(9).Signals(9).XData = [0 20.05 20.05 100]
      | sbobj.Groups(9).Signals(9).YData = [8 8 3 3]
      | sbobj.Groups(9).Signals(10).Name = 'state_FuelPriRelay'
      | sbobj.Groups(9).Signals(10).XData = [0 20.5 100]
      | sbobj.Groups(9).Signals(10).YData = [8 8 8]
      | sbobj.Groups(10).Name = 'NONFUNC'
      | sbobj.Groups(10).Signals(1).Name = 'dfbk_FuelPriOutput'
      | sbobj.Groups(10).Signals(1).XData = [0 20 20 22.2 22.2 60 60 61.4 61.4 100]
      | sbobj.Groups(10).Signals(1).YData = [0 0 1 1 0 0 1 1 0 0]
      | sbobj.Groups(10).Signals(2).Name = 'din_FuelPriRelay'
      | sbobj.Groups(10).Signals(2).XData = [0 20 20 22.2 22.2 60 60 61.4 61.4 100]
      | sbobj.Groups(10).Signals(2).YData = [0 0 1 1 0 0 1 1 0 0]
      | sbobj.Groups(10).Signals(3).Name = 'error_FuelSec'
      | sbobj.Groups(10).Signals(3).XData = [0 100]
      | sbobj.Groups(10).Signals(3).YData = [8 8]
      | sbobj.Groups(10).Signals(4).Name = 'state_Engine'
      | sbobj.Groups(10).Signals(4).XData = [0 20 20 30 30 50 50 60 60 61.2 61.2 62.6 62.6 64.2 64.2 100]
      | sbobj.Groups(10).Signals(4).YData = [1 1 2 2 3 3 1 1 2 2 1 1 2 2 1 1]
      | sbobj.Groups(10).Signals(5).Name = 'flt_ECT'
      | sbobj.Groups(10).Signals(5).XData = [0 49.9 49.9 100]
      | sbobj.Groups(10).Signals(5).YData = [0 0 200 200]
      | sbobj.Groups(10).Signals(6).Name = 'timer_Resolution'
      | sbobj.Groups(10).Signals(6).XData = [0 100]
      | sbobj.Groups(10).Signals(6).YData = [0 0]
      | sbobj.Groups(10).Signals(7).Name = 'state_Battery'
      | sbobj.Groups(10).Signals(7).XData = [0 100]
      | sbobj.Groups(10).Signals(7).YData = [8 8]
      | sbobj.Groups(10).Signals(8).Name = 'dout_FuelPrimary'
      | sbobj.Groups(10).Signals(8).XData = [0 20 60 100]
      | sbobj.Groups(10).Signals(8).YData = [0 0 0 0]
      | sbobj.Groups(10).Signals(9).Name = 'state_FuelPriOutput'
      | sbobj.Groups(10).Signals(9).XData = [0 100]
      | sbobj.Groups(10).Signals(9).YData = [8 8]
      | sbobj.Groups(10).Signals(10).Name = 'state_FuelPriRelay'
      | sbobj.Groups(10).Signals(10).XData = [0 100]
      | sbobj.Groups(10).Signals(10).YData = [8 8]
      | sbobj.Groups(11).Name = 'NO FDBK'
      | sbobj.Groups(11).Signals(1).Name = 'dfbk_FuelPriOutput'
      | sbobj.Groups(11).Signals(1).XData = [0 100]
      | sbobj.Groups(11).Signals(1).YData = [0 0]
      | sbobj.Groups(11).Signals(2).Name = 'din_FuelPriRelay'
      | sbobj.Groups(11).Signals(2).XData = [0 20 20 20.6 20.6 100]
      | sbobj.Groups(11).Signals(2).YData = [0 0 1 1 0 0]
      | sbobj.Groups(11).Signals(3).Name = 'error_FuelSec'
      | sbobj.Groups(11).Signals(3).XData = [0 100]
      | sbobj.Groups(11).Signals(3).YData = [8 8]
      | sbobj.Groups(11).Signals(4).Name = 'state_Engine'
      | sbobj.Groups(11).Signals(4).XData = [0 20 20 30 30 50 50 100]
      | sbobj.Groups(11).Signals(4).YData = [1 1 2 2 3 3 1 1]
      | sbobj.Groups(11).Signals(5).Name = 'flt_ECT'
      | sbobj.Groups(11).Signals(5).XData = [0 100]
      | sbobj.Groups(11).Signals(5).YData = [130 130]
      | sbobj.Groups(11).Signals(6).Name = 'timer_Resolution'
      | sbobj.Groups(11).Signals(6).XData = [0 100]
      | sbobj.Groups(11).Signals(6).YData = [0 0]
      | sbobj.Groups(11).Signals(7).Name = 'state_Battery'
      | sbobj.Groups(11).Signals(7).XData = [0 100]
      | sbobj.Groups(11).Signals(7).YData = [8 8]
      | sbobj.Groups(11).Signals(8).Name = 'dout_FuelPrimary'
      | sbobj.Groups(11).Signals(8).XData = [0 20 20 21.61 21.61 100]
      | sbobj.Groups(11).Signals(8).YData = [0 0 1 1 0 0]
      | sbobj.Groups(11).Signals(9).Name = 'state_FuelPriOutput'
      | sbobj.Groups(11).Signals(9).XData = [0 20.5 100]
      | sbobj.Groups(11).Signals(9).YData = [8 8 8]
      | sbobj.Groups(11).Signals(10).Name = 'state_FuelPriRelay'
      | sbobj.Groups(11).Signals(10).XData = [0 100]
      | sbobj.Groups(11).Signals(10).YData = [8 8]
      | sbobj.Groups(12).Name = 'Output Error On'
      | sbobj.Groups(12).Signals(1).Name = 'dfbk_FuelPriOutput'
      | sbobj.Groups(12).Signals(1).XData = [0 20 20 50.2 50.2 60 60 61.4 61.4 100]
      | sbobj.Groups(12).Signals(1).YData = [0 0 1 1 0 0 1 1 0 0]
      | sbobj.Groups(12).Signals(2).Name = 'din_FuelPriRelay'
      | sbobj.Groups(12).Signals(2).XData = [0 20 20 49.9 49.9 60 60 61.4 61.4 100]
      | sbobj.Groups(12).Signals(2).YData = [0 0 1 1 0 0 1 1 0 0]
      | sbobj.Groups(12).Signals(3).Name = 'error_FuelSec'
      | sbobj.Groups(12).Signals(3).XData = [0 100]
      | sbobj.Groups(12).Signals(3).YData = [8 8]
      | sbobj.Groups(12).Signals(4).Name = 'state_Engine'
      | sbobj.Groups(12).Signals(4).XData = [0 100]
      | sbobj.Groups(12).Signals(4).YData = [1 1]
      | sbobj.Groups(12).Signals(5).Name = 'flt_ECT'
      | sbobj.Groups(12).Signals(5).XData = [0 49.9 49.9 100]
      | sbobj.Groups(12).Signals(5).YData = [0 0 200 200]
      | sbobj.Groups(12).Signals(6).Name = 'timer_Resolution'
      | sbobj.Groups(12).Signals(6).XData = [0 100]
      | sbobj.Groups(12).Signals(6).YData = [0 0]
      | sbobj.Groups(12).Signals(7).Name = 'state_Battery'
      | sbobj.Groups(12).Signals(7).XData = [0 100]
      | sbobj.Groups(12).Signals(7).YData = [8 8]
      | sbobj.Groups(12).Signals(8).Name = 'dout_FuelPrimary'
      | sbobj.Groups(12).Signals(8).XData = [0 20 100]
      | sbobj.Groups(12).Signals(8).YData = [0 0 0]
      | sbobj.Groups(12).Signals(9).Name = 'state_FuelPriOutput'
      | sbobj.Groups(12).Signals(9).XData = [0 20.51 20.51 100]
      | sbobj.Groups(12).Signals(9).YData = [8 8 2 2]
      | sbobj.Groups(12).Signals(10).Name = 'state_FuelPriRelay'
      | sbobj.Groups(12).Signals(10).XData = [0 100]
      | sbobj.Groups(12).Signals(10).YData = [8 8]
      | sbobj.Groups(13).Name = 'Output Error Off'
      | sbobj.Groups(13).Signals(1).Name = 'dfbk_FuelPriOutput'
      | sbobj.Groups(13).Signals(1).XData = [0 20 100]
      | sbobj.Groups(13).Signals(1).YData = [0 0 0]
      | sbobj.Groups(13).Signals(2).Name = 'din_FuelPriRelay'
      | sbobj.Groups(13).Signals(2).XData = [0 100]
      | sbobj.Groups(13).Signals(2).YData = [0 0]
      | sbobj.Groups(13).Signals(3).Name = 'error_FuelSec'
      | sbobj.Groups(13).Signals(3).XData = [0 100]
      | sbobj.Groups(13).Signals(3).YData = [8 8]
      | sbobj.Groups(13).Signals(4).Name = 'state_Engine'
      | sbobj.Groups(13).Signals(4).XData = [0 20 20 30 30 50 50 60 60 61.2 61.2 62.6 62.6 64.2 64.2 100]
      | sbobj.Groups(13).Signals(4).YData = [1 1 2 2 3 3 1 1 2 2 1 1 2 2 1 1]
      | sbobj.Groups(13).Signals(5).Name = 'flt_ECT'
      | sbobj.Groups(13).Signals(5).XData = [0 49.9 49.9 100]
      | sbobj.Groups(13).Signals(5).YData = [0 0 200 200]
      | sbobj.Groups(13).Signals(6).Name = 'timer_Resolution'
      | sbobj.Groups(13).Signals(6).XData = [0 100]
      | sbobj.Groups(13).Signals(6).YData = [0 0]
      | sbobj.Groups(13).Signals(7).Name = 'state_Battery'
      | sbobj.Groups(13).Signals(7).XData = [0 100]
      | sbobj.Groups(13).Signals(7).YData = [8 8]
      | sbobj.Groups(13).Signals(8).Name = 'dout_FuelPrimary'
      | sbobj.Groups(13).Signals(8).XData = [0 20 20 20.06 20.06 100]
      | sbobj.Groups(13).Signals(8).YData = [0 0 1 1 0 0]
      | sbobj.Groups(13).Signals(9).Name = 'state_FuelPriOutput'
      | sbobj.Groups(13).Signals(9).XData = [0 20.05 20.05 100]
      | sbobj.Groups(13).Signals(9).YData = [8 8 3 3]
      | sbobj.Groups(13).Signals(10).Name = 'state_FuelPriRelay'
      | sbobj.Groups(13).Signals(10).XData = [0 100]
      | sbobj.Groups(13).Signals(10).YData = [8 8]
  dfbk_FuelPriOutput : Outport  Tag=STV Outport
  din_FuelPriRelay : Outport  Tag=STV Outport  Port=2
  error_FuelSec : Outport  Tag=STV Outport  Port=3
  state_Engine : Outport  Tag=STV Outport  Port=4
  flt_ECT : Outport  Tag=STV Outport  Port=5
  timer_Resolution : Outport  Tag=STV Outport  Port=6
  state_Battery : Outport  Tag=STV Outport  Port=7
  dout_FuelPrimary : Outport  Tag=STV Outport  Port=8
  state_FuelPriOutput : Outport  Tag=STV Outport  Port=9
  state_FuelPriRelay : Outport  Tag=STV Outport  Port=10
  wires:
  FromWs/1 -> Demux/1
  Demux/1 -> dfbk_FuelPriOutput/1
  Demux/2 -> din_FuelPriRelay/1
  Demux/3 -> error_FuelSec/1
  Demux/4 -> state_Engine/1
  Demux/5 -> flt_ECT/1
  Demux/6 -> timer_Resolution/1
  Demux/7 -> state_Battery/1
  Demux/8 -> dout_FuelPrimary/1
  Demux/9 -> state_FuelPriOutput/1
  Demux/10 -> state_FuelPriRelay/1

== stateflow chart Fuel_Primary_Relay/RelaySolenoid ==
  state INACTIVE
    en:dout_FuelPri = INACTIVE;
  state ACTIVE
    en:dout_FuelPri = ACTIVE;
    du:FuelTiming();
  state INACTIVE_OFF
    en:dout_FuelPri = INACTIVE;
  state FuelTiming [function]
    (default) -> (junction 8)
    (junction 8) -> (junction 9) [order 1] : [(PullTime != UNLIMITED)...
        | && ((CD_FUEL_PRIMARY_ON_SECONDARY_FAILURE == NON_FUNCTIONAL) || (error_FuelSec == NORMAL))]
    (junction 8) -> (junction 10) [order 2]
    (junction 9) -> (junction 11) : {
        | outputTimer++;
        | }
    (junction 11) -> (junction 10)
  note: Failure still allows operation of the machine, the internal feedback doesn't work
      | but we still have the relay feedback to guild us.
  (default) -> INACTIVE
  INACTIVE_OFF -> INACTIVE : [(state_Engine == ENGINE_NOT_RUNNING)]
  ACTIVE -> INACTIVE [order 2] : [(state_Engine == ENGINE_NOT_RUNNING)]
  INACTIVE -> ACTIVE : [(CD_FUEL_PRIMARY_FUNCTION != NON_FUNCTIONAL)...
      | && (timer_Resolution == INACTIVE)...
      | && (state_Engine == ENGINE_CRANKING)...
      | && ((state_OutputError == NORMAL) || (state_OutputError == FAILURE))...
      | && (state_RelayError == NORMAL)]
      | {
      | outputTimer = 0;
      | }
  ACTIVE -> INACTIVE_OFF [order 1] : [(outputTimer >= PullTime)...
      | || !((state_OutputError == NORMAL) || (state_OutputError == FAILURE))...
      | || (state_RelayError != NORMAL)]
  data: dout_FuelPri output boolean; CD_FUEL_PRIMARY_FUNCTION parameter uint8; CD_FUEL_PRIMARY_ON_SECONDARY_FAILURE parameter uint8; state_OutputError input uint8; state_RelayError input uint8; outputTimer local uint16 =0; timer_Resolution input uint8 =0; error_FuelSec input double; state_Engine input uint8; UNLIMITED parameter uint16 =65535; ENGINE_NOT_RUNNING parameter uint8 =1; ACTIVE parameter uint8 =1; ENGINE_CRANKING parameter uint8 =2; INACTIVE parameter uint8 =1; NORMAL parameter uint8 =1; PullTime input uint16; NON_FUNCTIONAL parameter uint8; FAILURE parameter uint8
